simulink model "vienna_car_part3"  (R2019b)
settings: Solver=ode23t  StartTime=0.0  StopTime=100  MaxStep=1e-4  RelTol=1e-4
values from neighbouring files (symbols this model uses):
  integral_constant = 200    [main.m]
  proportinal_constat = 20    [main.m]
  simulation_length_track = track2_length    [main.m]
  slope_of_track = 0    [main.m]
undefined symbols (not defined in the file or in its folder): air_density, drag_coefficient, equ_mass_of_rot_parts, gravity, mass, rolling_resistance_coefficient_0, rolling_resistance_coefficient_1, surface_area, wheel_radius
libraries: simulink x1
settings Model: Creator=jamil  LastModifiedBy=jamil
settings SolverCC: ZeroCrossAlgorithm=Adaptive
settings DebuggingCC: IgnoredZcDiagnostic=none

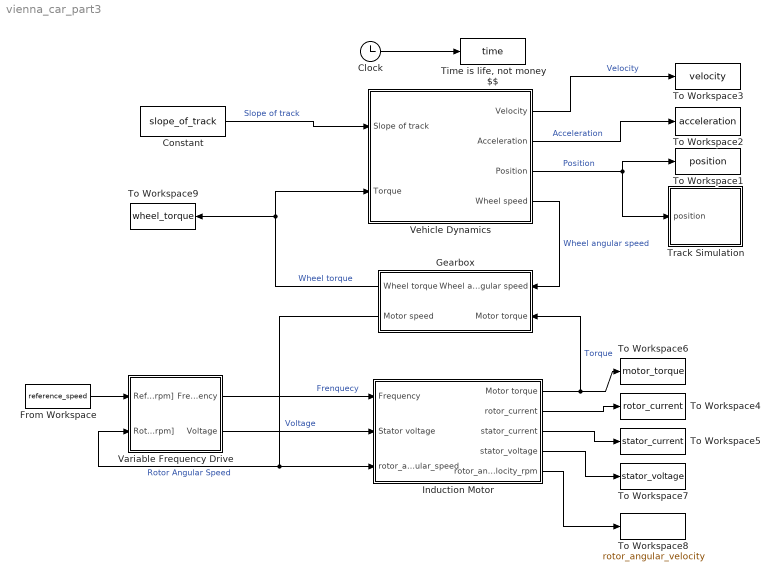
== system vienna_car_part3 ==
  Clock : Clock
  Constant : Constant  Value=slope_of_track
  From Workspace : FromWorkspace  VariableName=reference_speed  SampleTime=0
  Gearbox : Subsystem
      mask Display: image('pics/gearbox_pic.jpg'); % Use "Edit Image" on toolstrip to change.
  Induction Motor : Subsystem
      mask Display: image('pics/induction_motor_pic.jpg')
  "Time is life, not money $$" : ToWorkspace  VariableName=time  SampleTime=-1
  To Workspace1 : ToWorkspace  VariableName=position  SampleTime=-1
  To Workspace2 : ToWorkspace  VariableName=acceleration  SampleTime=-1
  To Workspace3 : ToWorkspace  VariableName=velocity  SampleTime=-1
  To Workspace4 : ToWorkspace  VariableName=rotor_current  SampleTime=-1
  To Workspace5 : ToWorkspace  VariableName=stator_current  SampleTime=-1
  To Workspace6 : ToWorkspace  VariableName=motor_torque  SampleTime=-1
  To Workspace7 : ToWorkspace  VariableName=stator_voltage  SampleTime=-1
  To Workspace8 : ToWorkspace  VariableName=rotor_angular_velocity  SampleTime=-1
  To Workspace9 : ToWorkspace  VariableName=wheel_torque  SampleTime=-1
  Track Simulation : Subsystem
  Variable Frequency Drive : Subsystem
      mask Display: image('pics/variable_speed_drive_pic.png')
  Vehicle Dynamics : Subsystem
      mask Display: image('pics/car_dynamic_pic.jpg'); % Use "Edit Image" on toolstrip to change.
  wires:
  Vehicle Dynamics/2(Acceleration) -> To Workspace2/1  "Acceleration"
  Vehicle Dynamics/3(Position) -> Track Simulation/1(position), To Workspace1/1  "Position"
  Constant/1 -> Vehicle Dynamics/1("Slope of track ")  "Slope of track"
  Vehicle Dynamics/1(Velocity) -> To Workspace3/1  "Velocity"
  Clock/1 -> "Time is life, not money $$"/1
  Gearbox/2(Motor speed) -> Variable Frequency Drive/2(Rotor Speed [rpm]), Induction Motor/3("rotor_angular_speed ")  "Rotor Angular Speed"
  Induction Motor/1(Motor torque) -> Gearbox/2(Motor torque), To Workspace6/1  "Torque"
  Variable Frequency Drive/1(Frequency) -> Induction Motor/1("Frequency ")  "Frenquecy"
  Variable Frequency Drive/2(Voltage) -> Induction Motor/2("Stator voltage ")  "Voltage"
  From Workspace/1 -> Variable Frequency Drive/1(Reference Speed [rpm])
  Induction Motor/4(stator_voltage) -> To Workspace7/1
  Induction Motor/5(rotor_angular_velocity_rpm) -> To Workspace8/1
  Induction Motor/2(rotor_current) -> To Workspace4/1
  Induction Motor/3(stator_current) -> To Workspace5/1
  Vehicle Dynamics/4(Wheel speed) -> Gearbox/1(Wheel angular speed)  "Wheel angular speed"
  Gearbox/1("Wheel torque ") -> To Workspace9/1, Vehicle Dynamics/2(Torque)  "Wheel torque"

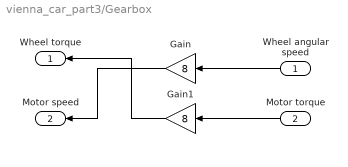
== system vienna_car_part3/Gearbox ==
  Wheel angular speed : Inport
  Motor torque : Inport  Port=2
  Gain : Gain  Gain=8
  Gain1 : Gain  Gain=8
  "Wheel torque " : Outport
  Motor speed : Outport  Port=2
  wires:
  Gain/1 -> Motor speed/1
  Wheel angular speed/1 -> Gain/1
  Gain1/1 -> "Wheel torque "/1
  Motor torque/1 -> Gain1/1

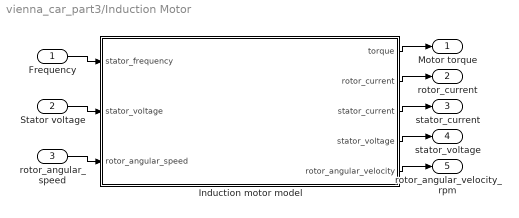
== system vienna_car_part3/Induction Motor ==
  "Frequency " : Inport
  "Stator voltage " : Inport  Port=2
  "rotor_angular_speed " : Inport  Port=3
  "Induction motor model " : MATLAB Function  TreatAsAtomicUnit=on
  Motor torque : Outport
  rotor_current : Outport  Port=2
  stator_current : Outport  Port=3
  stator_voltage : Outport  Port=4
  rotor_angular_velocity_rpm : Outport  Port=5
  wires:
  "Induction motor model "/1(torque) -> Motor torque/1
  "Stator voltage "/1 -> "Induction motor model "/2("stator_voltage ")
  "rotor_angular_speed "/1 -> "Induction motor model "/3(rotor_angular_speed)
  "Induction motor model "/2(rotor_current) -> rotor_current/1
  "Induction motor model "/3(stator_current) -> stator_current/1
  "Induction motor model "/4(stator_voltage) -> stator_voltage/1
  "Frequency "/1 -> "Induction motor model "/1(stator_frequency)
  "Induction motor model "/5(rotor_angular_velocity) -> rotor_angular_velocity_rpm/1

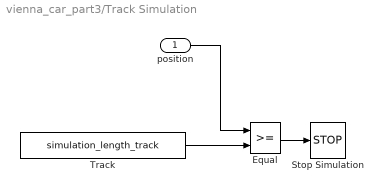
== system vienna_car_part3/Track Simulation ==
  position : Inport
  Equal : RelationalOperator  OutDataTypeStr=boolean  RndMeth=Simplest
  Stop Simulation : Stop
  "Track " : Constant  Value=simulation_length_track
  wires:
  Equal/1 -> Stop Simulation/1
  position/1 -> Equal/1
  "Track "/1 -> Equal/2

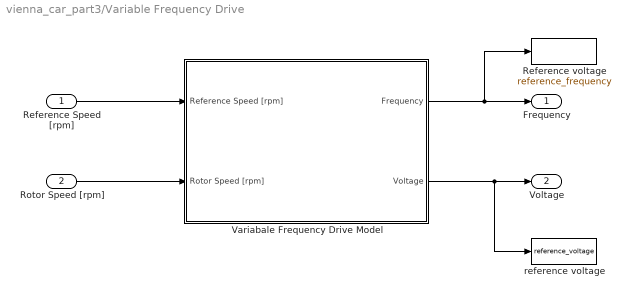
== system vienna_car_part3/Variable Frequency Drive ==
  Reference Speed [rpm] : Inport
  Rotor Speed [rpm] : Inport  Port=2
  Reference voltage : ToWorkspace  VariableName=reference_frequency  SampleTime=-1
  Variabale Frequency Drive Model : Subsystem
      mask Display: image('pics/variable_speed_drive_model.jpg')
  reference voltage : ToWorkspace  VariableName=reference_voltage  SampleTime=-1
  Frequency : Outport
  Voltage : Outport  Port=2
  wires:
  Variabale Frequency Drive Model/1(Frequency) -> Frequency/1, Reference voltage/1
  Variabale Frequency Drive Model/2(Voltage) -> Voltage/1, reference voltage/1
  Reference Speed [rpm]/1 -> Variabale Frequency Drive Model/1(Reference Speed [rpm])
  Rotor Speed [rpm]/1 -> Variabale Frequency Drive Model/2("Rotor Speed [rpm] ")

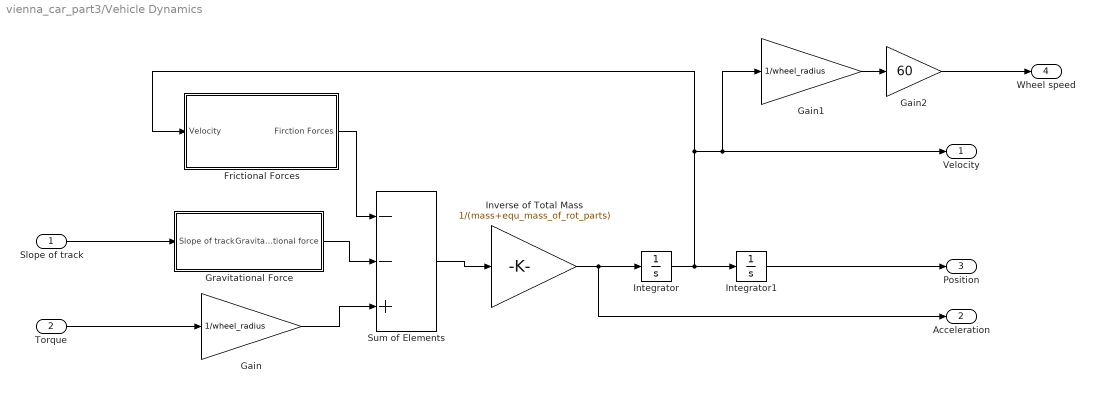
== system vienna_car_part3/Vehicle Dynamics ==
  "Slope of track " : Inport
  Torque : Inport  Port=2
  Frictional Forces : Subsystem
  Gain : Gain  Gain=1/wheel_radius
  Gain1 : Gain  Gain=1/wheel_radius
  Gain2 : Gain  Gain=60
  Gravitational Force : Subsystem
  Integrator : Integrator
  Integrator1 : Integrator
  Inverse of Total Mass : Gain  Gain=1/(mass+equ_mass_of_rot_parts)
  Sum of Elements : Sum  Inputs=--+
  Velocity : Outport
  Acceleration : Outport  Port=2
  Position : Outport  Port=3
  Wheel speed : Outport  Port=4
  wires:
  Integrator1/1 -> Position/1
  Inverse of Total Mass/1 -> Integrator/1, Acceleration/1
  Sum of Elements/1 -> Inverse of Total Mass/1
  Frictional Forces/1(Firction Forces) -> Sum of Elements/1
  "Slope of track "/1 -> Gravitational Force/1(Slope of track)
  Gravitational Force/1(Gravitational force) -> Sum of Elements/2
  Torque/1 -> Gain/1
  Gain/1 -> Sum of Elements/3
  Gain2/1 -> Wheel speed/1
  Integrator/1 -> Frictional Forces/1(Velocity), Gain1/1, Velocity/1, Integrator1/1
  Gain1/1 -> Gain2/1

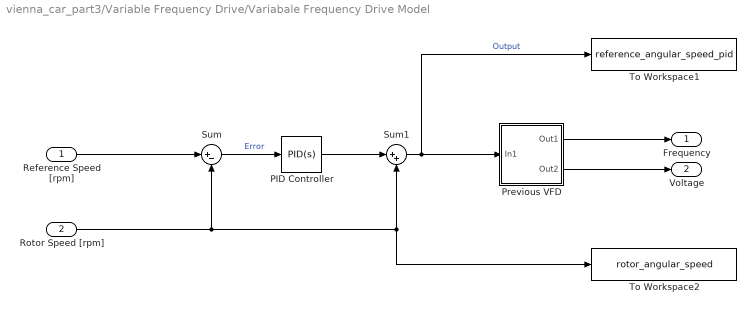
== system vienna_car_part3/Variable Frequency Drive/Variabale Frequency Drive Model ==
  Reference Speed [rpm] : Inport
  "Rotor Speed [rpm] " : Inport  Port=2
  PID Controller : simulink/Continuous/PID Controller  Controller=PID  Form=Parallel  TimeDomain=Continuous-time  SampleTime=-1  IntegratorMethod=Forward Euler  FilterMethod=Forward Euler  ControllerParametersSource=internal  P=proportinal_constat  I=integral_constant  D=0  UseFilter=on  N=100  TunerSelectOption=Transfer Function Based (PID Tuner App)  InitialConditionSource=internal  InitialConditionForIntegrator=0  InitialConditionForFilter=0  DifferentiatorICPrevScaledInput=0  ExternalReset=none  TrackingMode=off  Kt=1  LimitOutput=off  UpperSaturationLimit=inf  LowerSaturationLimit=-inf  LinearizeAsGain=on  AntiWindupMode=none  Kb=1  POutMin=[]  POutMax=[]  IOutMin=[]  IOutMax=[]  DOutMin=[]  DOutMax=[]  NOutMin=[]  NOutMax=[]  SumOutMin=[]  SumOutMax=[]  SaturationOutMin=[]  SaturationOutMax=[]  PParamMin=[]  PParamMax=[]  IParamMin=[]  IParamMax=[]  DParamMin=[]  DParamMax=[]  NParamMin=[]  NParamMax=[]  KbParamMin=[]  KbParamMax=[]  KtParamMin=[]  KtParamMax=[]  KbOutMin=[]  KbOutMax=[]  KtOutMin=[]  KtOutMax=[]  IntegratorOutMin=[]  IntegratorOutMax=[]  FilterOutMin=[]  FilterOutMax=[]  SumI1OutMin=[]  SumI1OutMax=[]  SumI2OutMin=[]  SumI2OutMax=[]  SumI3OutMin=[]  SumI3OutMax=[]  SumI4OutMin=[]  SumI4OutMax=[]  SumDOutMin=[]  SumDOutMax=[]  DifferentiatorOutMin=[]  DifferentiatorOutMax=[]  FilterDiffOutCoefMin=[]  FilterDiffOutCoefMax=[]  ReciprocalOutMin=[]  ReciprocalOutMax=[]  SumDenOutMin=[]  SumDenOutMax=[]  SumNumOutMin=[]  SumNumOutMax=[]  DivideOutMin=[]  DivideOutMax=[]  IntegratorContinuousStateAttributes=''  IntegratorStateMustResolveToSignalObject=off  IntegratorRTWStateStorageClass=Auto  FilterContinuousStateAttributes=''  FilterStateMustResolveToSignalObject=off  FilterRTWStateStorageClass=Auto  ParallelPVariant=InternalParameters  IdealPVariant=Disabled  IVariant=InternalParameters  DVariant=InternalParameters  IntegratorVariant=Continuous  SatVariant=Disabled  AWVariant=Passthrough  PCopyVariant=Disabled  TRVariant=Disabled  FdbkBlocksVariant=Forward  IdealPFdbkVariant=Disabled  SatFdbkVariant=Disabled  DerivativeFilterVariant=ContFilter  NVariant=InternalParameters  NCopyVariant=Disabled  FilterICVariant=InternalICsFilter  IntegratorICVariant=InternalICs  ExternalResetVariant=Disabled  TRSumVariant=Passthrough  SumFdbkVariant=Disabled  SumVariant=Sum_PID
  Previous VFD : Subsystem
  Sum : Sum  Inputs=|+-
  Sum1 : Sum  Inputs=|++
  To Workspace1 : ToWorkspace  VariableName=reference_angular_speed_pid  SampleTime=-1
  To Workspace2 : ToWorkspace  VariableName=rotor_angular_speed  SampleTime=-1
  Frequency : Outport
  Voltage : Outport  Port=2
  wires:
  "Rotor Speed [rpm] "/1 -> To Workspace2/1, Sum1/2, Sum/2
  Sum/1 -> PID Controller/1  "Error"
  PID Controller/1 -> Sum1/1
  Sum1/1 -> To Workspace1/1, Previous VFD/1(In1)  "Output"
  Previous VFD/1(Out1) -> Frequency/1
  Previous VFD/2(Out2) -> Voltage/1
  Reference Speed [rpm]/1 -> Sum/1

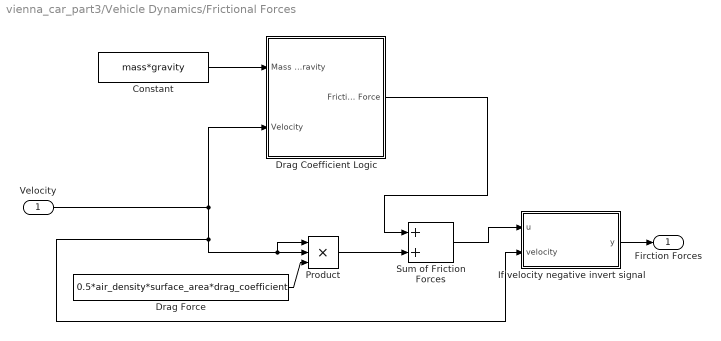
== system vienna_car_part3/Vehicle Dynamics/Frictional Forces ==
  Velocity : Inport
  Constant : Constant  Value=mass*gravity
  Drag Coefficient Logic : Subsystem
  Drag Force : Constant  Value=0.5*air_density*surface_area*drag_coefficient
  If velocity negative invert signal : MATLAB Function  TreatAsAtomicUnit=on
  Product : Product  Inputs=3
  Sum of Friction Forces : Sum
  Firction Forces : Outport
  wires:
  Drag Force/1 -> Product/3
  Constant/1 -> Drag Coefficient Logic/1("Mass and Gravity ")
  Drag Coefficient Logic/1(Friction Force) -> Sum of Friction Forces/1
  Velocity/1 -> Product/1, Product/2, If velocity negative invert signal/2(velocity), Drag Coefficient Logic/2(Velocity)
  Product/1 -> Sum of Friction Forces/2
  Sum of Friction Forces/1 -> If velocity negative invert signal/1(u)
  If velocity negative invert signal/1(y) -> Firction Forces/1

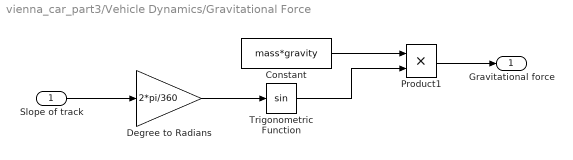
== system vienna_car_part3/Vehicle Dynamics/Gravitational Force ==
  Slope of track : Inport
  Constant : Constant  Value=mass*gravity
  Degree to Radians : Gain  Gain=2*pi/360
  Product1 : Product
  Trigonometric Function : Trigonometry
  Gravitational force : Outport
  wires:
  Product1/1 -> Gravitational force/1
  Constant/1 -> Product1/1
  Trigonometric Function/1 -> Product1/2
  Slope of track/1 -> Degree to Radians/1
  Degree to Radians/1 -> Trigonometric Function/1

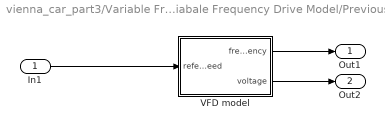
== system vienna_car_part3/Variable Frequency Drive/Variabale Frequency Drive Model/Previous VFD ==
  In1 : Inport
  VFD model : MATLAB Function  TreatAsAtomicUnit=on
  Out1 : Outport
  Out2 : Outport  Port=2
  wires:
  In1/1 -> VFD model/1(reference_speed)
  VFD model/2(voltage) -> Out2/1
  VFD model/1(frequency) -> Out1/1

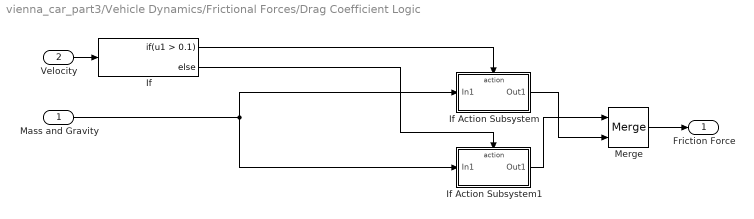
== system vienna_car_part3/Vehicle Dynamics/Frictional Forces/Drag Coefficient Logic ==
  "Mass and Gravity " : Inport
  Velocity : Inport  Port=2
  If : If  IfExpression=u1 > 0.1
  If Action Subsystem : Subsystem  TreatAsAtomicUnit=on
  If Action Subsystem1 : Subsystem  TreatAsAtomicUnit=on
  Merge : Merge
  Friction Force : Outport
  wires:
  If Action Subsystem/1(Out1) -> Merge/2
  If Action Subsystem1/1(Out1) -> Merge/1
  If/2 -> If Action Subsystem1/Action
  "Mass and Gravity "/1 -> If Action Subsystem/1(In1), If Action Subsystem1/1(In1)
  Merge/1 -> Friction Force/1
  If/1 -> If Action Subsystem/Action
  Velocity/1 -> If/1

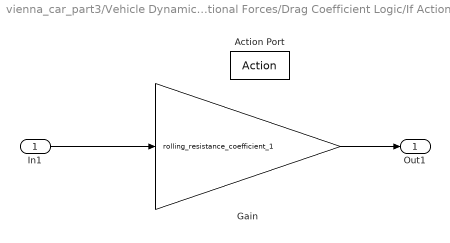
== system vienna_car_part3/Vehicle Dynamics/Frictional Forces/Drag Coefficient Logic/If Action Subsystem ==
  In1 : Inport
  Action Port : ActionPort  ActionPortLabel=if(u1 > 0.1)
  Gain : Gain  Gain=rolling_resistance_coefficient_1
  Out1 : Outport
  wires:
  In1/1 -> Gain/1
  Gain/1 -> Out1/1

== system vienna_car_part3/Vehicle Dynamics/Frictional Forces/Drag Coefficient Logic/If Action Subsystem1 ==
  In1 : Inport
  Action Port : ActionPort  ActionPortLabel=else
  Gain : Gain  Gain=rolling_resistance_coefficient_0
  Out1 : Outport
  wires:
  In1/1 -> Gain/1
  Gain/1 -> Out1/1

== matlab function vienna_car_part3/Variable Frequency Drive/Variabale Frequency Drive Model/Previous VFD/VFD model ==
  data: reference_speed input; frequency output; voltage output
function [frequency, voltage] = fcn(reference_speed)
frequency = (reference_speed*2)/60;
voltage = frequency;
end

== matlab function vienna_car_part3/Induction Motor/Induction motor model  ==
  data: stator_frequency input; torque output; stator_voltage input; rotor_angular_speed input; rotor_current output; stator_current output; stator_voltage output; rotor_angular_velocity output
function [torque, rotor_current, stator_current, stator_voltage, rotor_angular_velocity] = fcn(stator_frequency, stator_voltage, rotor_angular_speed)
    % slip
    if (rotor_angular_speed >= 0)
        slip = (60*stator_frequency/2 - rotor_angular_speed)/(60*stator_frequency/2); %rpm
    else
        slip = 1;
    end
    % Constant specs
    stator_resistance = 8.56*1e-3;
    stator_leakage_inductance = 0.06292 * 1e-3;
    mutual_inductance = 1.0122 * 1e-3;
    rotor_resistance = 10.20 *1e-3;
    rotor_leakage_inductance = 0.06709 * 1e-3;
    % Variable specs
    stator_voltage = stator_voltage/sqrt(3); % phase-phase -> % phase-neutral (rms value)
    stator_reactance = stator_leakage_inductance * 2 * pi * stator_frequency * 1i;
    rotor_reactance = rotor_leakage_inductance * 2 * pi * stator_frequency * 1i;
    mutual_reactance = mutual_inductance * 2 * pi * stator_frequency * 1i;
    stator_impedance = stator_resistance + stator_reactance; % 
    rotor_impedance = rotor_resistance + rotor_reactance; 
    % Descriptive Equations
    equivalent_impedance = stator_impedance + (mutual_reactance*(((-slip +1)/slip)*rotor_resistance+rotor_impedance))/(mutual_reactance+(((-slip+1)/slip)*rotor_resistance+rotor_impedance));
    stator_current = stator_voltage/equivalent_impedance;
     % Calculus of torque
     rotor_current = stator_current - (stator_voltage-stator_current*stator_impedance)/(mutual_reactance); %(already in rmsrms)
     if (slip == 0)
         torque = 0;
     else
         torque = (3*rotor_resistance*abs(rotor_current)^2)/(slip*stator_frequency*2*pi); %if s = 0 => binario  igual a 0
     end
     rotor_angular_velocity = (1-slip)*stator_frequency*60;
end
% power and torque -> need to calculate rms
% Look at the exression of the torque an put slip = 1 and look at the
% relation .TODO
% SOlver -> Predict next solutions and see if the error is big ... if it
% has a great diference ... if the signal has too much oscilations,
% decrease the step time in the solver

== matlab function vienna_car_part3/Vehicle Dynamics/Frictional Forces/If velocity negative invert signal ==
  data: u input; y output; velocity input
function y = fcn(u, velocity)
if (velocity < 0 )
    y = - u;
else
    y = u;
end
end
